simulink library "calcFluidDynamicLoadsUnpartitioned"  (R2020a)
settings: Solver=VariableStepAuto  StartTime=0.0  StopTime=10.0  RelTol=1e-3
undefined symbols (not defined in the file or in its folder): vhcl
libraries: vrlib x3, dynamicPressure_ul x1, eeGeneralControl x1, ctrlSurfCalc_cl x1, alphaBetaLE_ul x1, localApparentWind_ul x1, rotateAboutVec x1
settings Model: Creator=Ayaz  LastModifiedBy=adabney

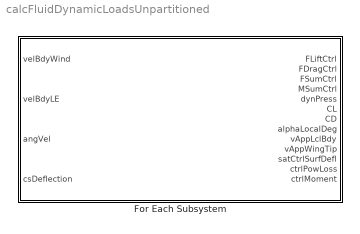
== system calcFluidDynamicLoadsUnpartitioned ==
  For Each Subsystem : Subsystem  TreatAsAtomicUnit=on  mask{aSurf=vhcl.struct('OCT.aeroSurf'), sRef=vhcl.fluidRefArea.Value}
      mask prompts: aSurf "Vehicle"; sRef "Reference Area"

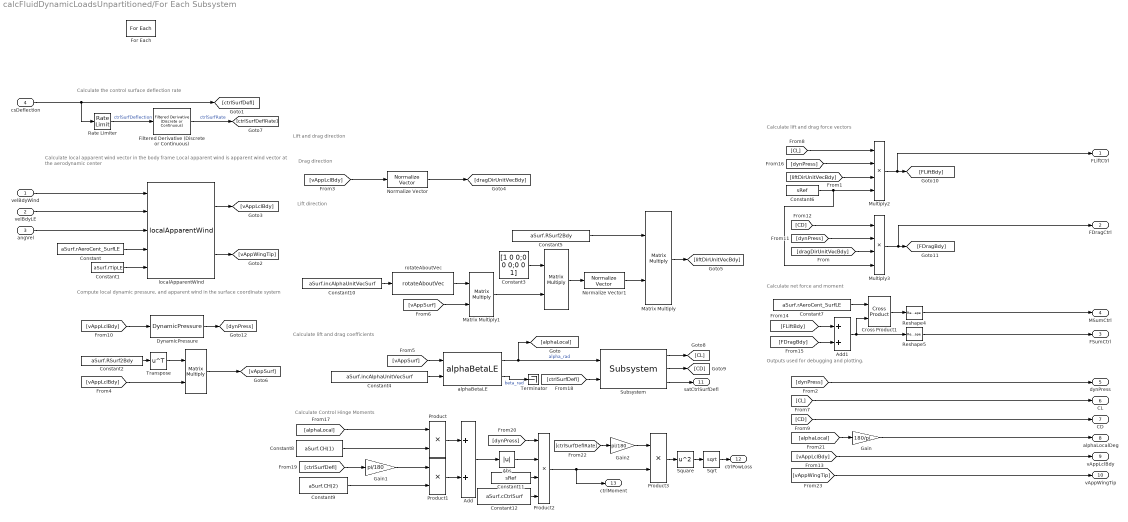
== system calcFluidDynamicLoadsUnpartitioned/For Each Subsystem ==
  note: Compute local dynamic pressure,
      | and apparent wind in the surface coordinate system
  note: Lift and drag direction
  note: Calculate Control Hinge Moments
  note: Drag direction
  note: Calculate lift and drag coefficients
  note: Calculate net force and moment
  note: Calculate the control surface deflection rate
  note: Outputs used for debugging and plotting.
  note: Lift direction
  note: Calculate lift and drag force vectors
  note: Calculate local apparent wind vector in the body frame
      | Local apparent wind is apparent wind vector at the aerodynamic center
  velBdyWind : Inport  Partition=on  PartitionDimension=2  PartitionWidth=1  PartitionOffset=0
  velBdyLE : Inport  Port=2
  angVel : Inport  Port=3
  csDeflection : Inport  Port=4  Partition=on  PartitionDimension=1  PartitionWidth=1  PartitionOffset=0
  " " : Product  Multiplication=Matrix(*)
  "  " : Product  Multiplication=Matrix(*)
  Abs : Abs
  Add : Sum
  Add1 : Sum
  Constant : Constant  Value=aSurf.rAeroCent_SurfLE  VectorParams1D=off
  Constant1 : Constant  Value=aSurf.rTipLE  VectorParams1D=off
  Constant10 : Constant  Value=aSurf.incAlphaUnitVecSurf  VectorParams1D=off
  Constant11 : Constant  Value=sRef
  Constant12 : Constant  Value=aSurf.cCtrlSurf
  Constant2 : Constant  Value=aSurf.RSurf2Bdy  VectorParams1D=off
  Constant3 : Constant  Value=[1 0 0;0 0 0;0 0 1]  VectorParams1D=off
  Constant4 : Constant  Value=aSurf.incAlphaUnitVecSurf  VectorParams1D=off
  Constant5 : Constant  Value=aSurf.RSurf2Bdy  VectorParams1D=off
  Constant6 : Constant  Value=sRef
  Constant7 : Constant  Value=aSurf.rAeroCent_SurfLE  VectorParams1D=off
  Constant8 : Constant  Value=aSurf.CH(1)
  Constant9 : Constant  Value=aSurf.CH(2)
  Cross Product1 : vrlib/Utilities/Cross Product
  DynamicPressure : dynamicPressure_ul/DynamicPressure  rho=fluidDensity
  Filtered Derivative (Discrete or Continuous) : eeGeneralControl/Filtered Derivative (Discrete or Continuous)  K=1  T=.001  B=inf  A=-inf  minRatio=10  init_option=Inherited from block input  x0=0  Ts=-1
      settings: SourceProductBaseCode=PS
  For Each : ForEach  DisableCoverage=on  IterateSubsysMaskParameter=on
  Gain : Gain  Gain=180/pi
  Gain1 : Gain  Gain=pi/180
  Gain2 : Gain  Gain=pi/180
  Matrix Multiply : Product  Multiplication=Matrix(*)
  Matrix Multiply1 : Product  Multiplication=Matrix(*)
  Multiply2 : Product  Inputs=4
  Multiply3 : Product  Inputs=4
  Normalize Vector : vrlib/Utilities/Normalize Vector  maxzero=0
  Normalize Vector1 : vrlib/Utilities/Normalize Vector  maxzero=0
  Product : Product
  Product1 : Product
  Product2 : Product  Inputs=4
  Product3 : Product
  Rate Limiter : RateLimiter  RisingSlewLimit=aSurf.maxCtrlDefSpeed.Value  FallingSlewLimit=-aSurf.maxCtrlDefSpeed.Value  SampleTimeMode=inherited
  Reshape4 : Reshape  OutputDimensionality=Column vector (2-D)
  Reshape5 : Reshape  OutputDimensionality=Column vector (2-D)
  Sqrt : Sqrt  SaturateOnIntegerOverflow=on
  Square : Math  Operator=square  SaturateOnIntegerOverflow=on
  Subsystem : ctrlSurfCalc_cl/Subsystem  aSurf=aSurf
  Terminator : Terminator
  Transpose : Math  Operator=transpose  SignedPower=on  SaturateOnIntegerOverflow=on
  alphaBetaLE : alphaBetaLE_ul/alphaBetaLE  SystemSampleTime=-1  Latency=0  AutoFrameSizeCalculation=off
  localApparentWind : localApparentWind_ul/localApparentWind  SystemSampleTime=-1  Latency=0  AutoFrameSizeCalculation=off
  rotateAboutVec : rotateAboutVec/rotateAboutVec  ang=90
  FLiftCtrl : Outport  ConcatenationDimension=1  VectorParamsAs1DForOutWhenUnconnected=off
  FDragCtrl : Outport  Port=2  ConcatenationDimension=1  VectorParamsAs1DForOutWhenUnconnected=off
  FSumCtrl : Outport  Port=3  ConcatenationDimension=1  VectorParamsAs1DForOutWhenUnconnected=off
  MSumCtrl : Outport  Port=4  PortDimensions=[3 1]  ConcatenationDimension=1  VectorParamsAs1DForOutWhenUnconnected=off
  dynPress : Outport  Port=5  ConcatenationDimension=1  VectorParamsAs1DForOutWhenUnconnected=off
  CL : Outport  Port=6  ConcatenationDimension=1  VectorParamsAs1DForOutWhenUnconnected=off
  CD : Outport  Port=7  ConcatenationDimension=1  VectorParamsAs1DForOutWhenUnconnected=off
  alphaLocalDeg : Outport  Port=8  ConcatenationDimension=1  VectorParamsAs1DForOutWhenUnconnected=off
  vAppLclBdy : Outport  Port=9  ConcatenationDimension=1  VectorParamsAs1DForOutWhenUnconnected=off
  vAppWingTip : Outport  Port=10  ConcatenationDimension=1  VectorParamsAs1DForOutWhenUnconnected=off
  satCtrlSurfDefl : Outport  Port=11  ConcatenationDimension=1
  ctrlPowLoss : Outport  Port=12  ConcatenationDimension=1
  ctrlMoment : Outport  Port=13  ConcatenationDimension=1
  wires:
  Subsystem/3 -> satCtrlSurfDefl/1
  alphaBetaLE/1 -> Subsystem/1, [alphaLocal]  "alpha_rad"
  Constant5/1 -> Matrix Multiply/1
  Subsystem/1 -> [CL]
  Subsystem/2 -> [CD]
  [ctrlSurfDefl] -> Subsystem/2
  "  "/1 -> [vAppSurf]
  [vAppLclBdy] -> DynamicPressure/1
  localApparentWind/2 -> [vAppWingTip]
  Constant1/1 -> localApparentWind/5
  Constant/1 -> localApparentWind/4
  DynamicPressure/1 -> [dynPress]
  [vAppLclBdy] -> "  "/2
  Constant4/1 -> alphaBetaLE/2
  velBdyWind/1 -> localApparentWind/1
  angVel/1 -> localApparentWind/3
  alphaBetaLE/2 -> Terminator/1  "beta_rad"
  Transpose/1 -> "  "/1
  Matrix Multiply1/1 -> " "/2
  Constant3/1 -> " "/1
  [vAppSurf] -> alphaBetaLE/1
  Constant6/1 -> Multiply2/4, Multiply3/4
  [vAppLclBdy] -> vAppLclBdy/1
  [vAppLclBdy] -> Normalize Vector/1
  [vAppSurf] -> Matrix Multiply1/2
  Abs/1 -> Product2/2
  Product3/1 -> Square/1
  [dynPress] -> dynPress/1
  Constant10/1 -> rotateAboutVec/1
  Constant11/1 -> Product2/3
  Sqrt/1 -> ctrlPowLoss/1
  Reshape5/1 -> FSumCtrl/1
  csDeflection/1 -> [ctrlSurfDefl], Rate Limiter/1
  [CD] -> CD/1
  Gain2/1 -> Product3/1
  " "/1 -> Normalize Vector1/1
  Gain1/1 -> Product1/1
  Rate Limiter/1 -> Filtered Derivative (Discrete or Continuous)/1  "ctrlSurfDeflection"
  Constant12/1 -> Product2/4
  [alphaLocal] -> Product/1
  Square/1 -> Sqrt/1
  Constant8/1 -> Product/2
  [dynPress] -> Product2/1
  [CD] -> Multiply3/1
  Matrix Multiply/1 -> [liftDirUnitVecBdy]
  [ctrlSurfDefl] -> Gain1/1
  Product/1 -> Add/1
  Cross Product1/1 -> Reshape4/1
  Reshape4/1 -> MSumCtrl/1
  [FDragBdy] -> Add1/2
  Product1/1 -> Add/2
  [liftDirUnitVecBdy] -> Multiply2/3
  rotateAboutVec/1 -> Matrix Multiply1/1
  [CL] -> CL/1
  Filtered Derivative (Discrete or Continuous)/1 -> [ctrlSurfDeflRate]  "ctrlSurfRate"
  Constant7/1 -> Cross Product1/1
  localApparentWind/1 -> [vAppLclBdy]
  Add1/1 -> Cross Product1/2, Reshape5/1
  Gain/1 -> alphaLocalDeg/1
  velBdyLE/1 -> localApparentWind/2
  [dragDirUnitVecBdy] -> Multiply3/3
  [dynPress] -> Multiply2/2
  Multiply2/1 -> [FLiftBdy], FLiftCtrl/1
  [CL] -> Multiply2/1
  [alphaLocal] -> Gain/1
  [dynPress] -> Multiply3/2
  [ctrlSurfDeflRate] -> Gain2/1
  Normalize Vector1/1 -> Matrix Multiply/2
  Add/1 -> Abs/1
  Constant2/1 -> Transpose/1
  Constant9/1 -> Product1/2
  Product2/1 -> ctrlMoment/1, Product3/2
  [FLiftBdy] -> Add1/1
  [vAppWingTip] -> vAppWingTip/1
  Normalize Vector/1 -> [dragDirUnitVecBdy]
  Multiply3/1 -> [FDragBdy], FDragCtrl/1
